simulink model "disturbo_n"  (R2022b)
settings: Solver=VariableStepAuto  StartTime=0.0  StopTime=10.0  RelTol=1e-3
model workspace (MAT data in the model file):
  amplitude_n = Simulink.Parameter
  amplitude_n.Value = 1
  amplitude_n.DataType = 'auto'
  amplitude_n.Complexity = 'real'
  amplitude_n.Dimensions = [1 1]
settings Model: ParameterArgumentNames=amplitude_n  Creator=eleon  LastModifiedBy=eleon

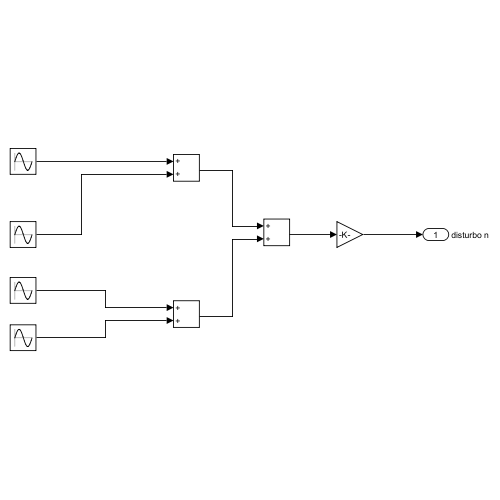
[thumbnail: Simulink's stored preview of the top-level diagram]
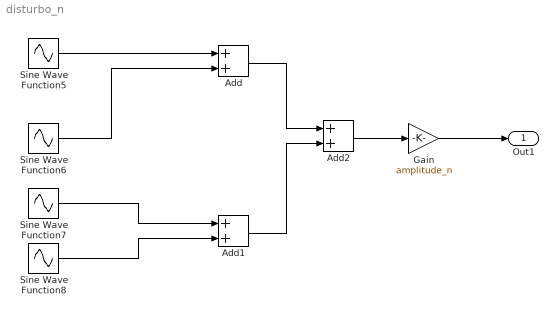
== system disturbo_n ==
  Add : Sum
  Add1 : Sum
  Add2 : Sum
  Gain : Gain  Gain=amplitude_n
  Sine Wave Function5 : Sin  Amplitude=0.6  Frequency=10^3  SampleTime=0
  Sine Wave Function6 : Sin  Amplitude=0.6  Frequency=10^3*2  SampleTime=0
  Sine Wave Function7 : Sin  Amplitude=0.6  Frequency=10^3*3  SampleTime=0
  Sine Wave Function8 : Sin  Amplitude=0.6  Frequency=10^3*4  SampleTime=0
  Out1 : Outport  SignalName=disturbo n
  wires:
  Sine Wave Function5/1 -> Add/1
  Sine Wave Function6/1 -> Add/2
  Add/1 -> Add2/1
  Add1/1 -> Add2/2
  Sine Wave Function7/1 -> Add1/1
  Sine Wave Function8/1 -> Add1/2
  Add2/1 -> Gain/1
  Gain/1 -> Out1/1
